simulink model "flightControlSystem"  (R2019b)
settings: Solver=ode3  StartTime=0  StopTime=TFinal  FixedStep=Ts  RelTol=1e-3  EnableMultiTasking=on
undefined symbols (not defined in the file): BINARIZER_THRESHOLD, codertarget, COG_X, COG_Y, Controller, DELAY_LANDING, DERIVATIVE_GAIN, DiscIntNeverNeededParam, Discrete, DISK_KERNEL, Estimator, FLAG_WAIT_FOR_HOVERING, FOV, FRAME_SIZE_HEIGHT, FRAME_SIZE_WIDTH, g, G_B_GAIN, GAIN_LANDING, GAIN_TRACK, gray, init, MAX_RADIUS_CROWN, MIN_RADIUS_CROWN, Sensors, SQUARE_KERNEL, strel, Time, TIME_HOLD, Ts, Vehicle, Z_HIGH, Z_LOW
libraries: simulink x37, sharedtransform x3, ctrlSharedLib x2, visionmorphops x2, sharedutil x1, parrotlib x1
(part 2 of 3)

== system flightControlSystem/Control System/Path Planning/Non linear Path Planner/Z PLANNER ==
  error_x : Inport
  flag_end_marker : Inport  Port=2
  error_y : Inport  Port=3
  flag_track : Inport  Port=4
  Chart : Stateflow chart  BlockKeywords=__PRM__SERIALIZED__DATA__:Stateflow Chart,Stateflow Diagram  TreatAsAtomicUnit=on
  Delay1 : Delay  DelayLength=DELAY_LANDING
  MATLAB Function : MATLAB Function  TreatAsAtomicUnit=on
  z_planned : Outport  VectorParamsAs1DForOutWhenUnconnected=off
  flag_end_marker_to_controller : Outport  Port=2  VectorParamsAs1DForOutWhenUnconnected=off
  wires:
  error_y/1 -> MATLAB Function/2(error_y)
  error_x/1 -> MATLAB Function/1(error_x)
  flag_end_marker/1 -> Chart/2(flag_end_marker), MATLAB Function/3(flag_end_marker)
  MATLAB Function/2(norm_error) -> Delay1/1
  Delay1/1 -> MATLAB Function/4(norm_error_prev)
  MATLAB Function/1(norm_error_tot) -> Chart/1(norm_error)
  Chart/1(z_planned) -> z_planned/1
  flag_track/1 -> Chart/3(flag_track)
  Chart/2(flag_end_marker_to_controller) -> flag_end_marker_to_controller/1

== system flightControlSystem/Control System/State Estimator/Complementary Filter/If Action Subsystem ==
  rpy : Inport
  accel : Inport  Port=2
  Action Port : ActionPort  ActionPortLabel=if(u1 > 0)
  Demux : Demux  Outputs=3
  Demux1 : Demux  Outputs=3
  Divide : Product  Inputs=*/
  Gain : Gain  Gain=1-Estimator.gyroAngleUpdateAccWeight
  Gain1 : Gain  Gain=Estimator.gyroAngleUpdateAccWeight
  Gain2 : Gain  Gain=1/g
  Gain3 : Gain  Gain=Estimator.gyroAngleUpdateAccWeight
  Gain4 : Gain  Gain=1-Estimator.gyroAngleUpdateAccWeight
  Mux : Mux  Inputs=2
  Sum : Sum  Inputs=|++
  Sum1 : Sum  Inputs=|++
  Terminator1 : Terminator
  Trigonometric Function : Trigonometry  Operator=atan
  Trigonometric Function1 : Trigonometry  Operator=asin
  pitch,roll : Outport  VectorParamsAs1DForOutWhenUnconnected=off
  wires:
  accel/1 -> Demux/1
  Demux/2 -> Divide/1
  Demux/3 -> Divide/2
  Divide/1 -> Trigonometric Function/1
  Gain/1 -> Sum/1
  Trigonometric Function/1 -> Gain1/1
  Mux/1 -> pitch,roll/1
  Gain2/1 -> Trigonometric Function1/1
  Trigonometric Function1/1 -> Gain3/1
  Gain4/1 -> Sum1/1
  Gain3/1 -> Sum1/2
  Sum1/1 -> Mux/1
  Sum/1 -> Mux/2
  rpy/1 -> Demux1/1
  Demux1/1 -> Gain/1
  Demux1/2 -> Gain4/1
  Demux/1 -> Gain2/1
  Demux1/3 -> Terminator1/1
  Gain1/1 -> Sum/2

== system flightControlSystem/Control System/State Estimator/Complementary Filter/If Action Subsystem2 ==
  prin : Inport
  Action Port : ActionPort  ActionPortLabel=else
  prout : Outport  VectorParamsAs1DForOutWhenUnconnected=off
  wires:
  prin/1 -> prout/1

== system flightControlSystem/Control System/State Estimator/Complementary Filter/Wbe ==
  rpy : Inport  OutDataTypeStr=single
  Constant : Constant  Value=single(0)
  Create 3x3 Matrix : sharedutil/Create 3x3 Matrix  aMode=aMode
  Divide : Product  Inputs=*/
  Gain : Gain  Gain=-1
  Product{1..4} (4 alike) : Product
  Selector : Selector  InputPortWidth=3  IndexOptions=Index vector (dialog)  Indices=[1]  OutputSizes=1
  Selector1 : Selector  InputPortWidth=3  IndexOptions=Index vector (dialog)  Indices=[1]  OutputSizes=1
  Selector2 : Selector  InputPortWidth=3  IndexOptions=Index vector (dialog)  Indices=[2]  OutputSizes=1
  Selector3 : Selector  InputPortWidth=3  IndexOptions=Index vector (dialog)  Indices=[2]  OutputSizes=1
  Trigonometric Function : Trigonometry  Operator=sincos
  Wbe : Outport  VectorParamsAs1DForOutWhenUnconnected=off
  wires:
  Create 3x3 Matrix/1 -> Divide/1
  Product3/1 -> Create 3x3 Matrix/8
  Trigonometric Function/2 -> Selector1/1, Selector2/1
  Selector3/1 -> Product4/2, Product3/2
  Selector1/1 -> Product4/1, Product1/1, Create 3x3 Matrix/3
  Trigonometric Function/1 -> Selector3/1, Selector/1
  Product1/1 -> Create 3x3 Matrix/5
  Product2/1 -> Create 3x3 Matrix/6
  Selector2/1 -> Divide/2, Create 3x3 Matrix/7, Product2/1, Product1/2
  Gain/1 -> Product2/2
  Product4/1 -> Create 3x3 Matrix/9
  Constant/1 -> Create 3x3 Matrix/4, Create 3x3 Matrix/1
  Divide/1 -> Wbe/1
  rpy/1 -> Trigonometric Function/1
  Selector/1 -> Product3/1, Gain/1, Create 3x3 Matrix/2

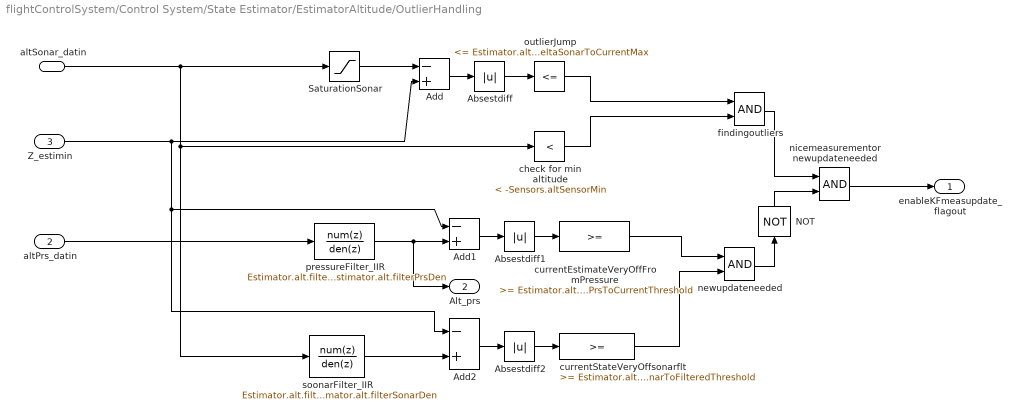
== system flightControlSystem/Control System/State Estimator/EstimatorAltitude/OutlierHandling ==
  altSonar_datin : Inport
  altPrs_datin : Inport  Port=2
  Z_estimin : Inport  Port=3
  Absestdiff : Abs
  Absestdiff1 : Abs
  Absestdiff2 : Abs
  Add : Sum  Inputs=-+
  Add1 : Sum  Inputs=-+
  Add2 : Sum  Inputs=-+
  NOT : Logic  Operator=NOT  IconShape=distinctive  AllPortsSameDT=off  OutDataTypeStr=boolean
  SaturationSonar : Saturate  UpperLimit=-Sensors.altSensorMin  LowerLimit=-inf
  check for min altitude : simulink/Logic and Bit Operations/Compare To Constant  relop=<  const=-Sensors.altSensorMin  OutDataTypeStr=boolean
  currentEstimateVeryOffFromPressure : simulink/Logic and Bit Operations/Compare To Constant  relop=>=  const=Estimator.alt.deltaPrsToCurrentThreshold  OutDataTypeStr=boolean
  currentStateVeryOffsonarflt : simulink/Logic and Bit Operations/Compare To Constant  relop=>=  const=Estimator.alt.deltaSonarToFilteredThreshold  OutDataTypeStr=boolean
  findingoutliers : Logic  AllPortsSameDT=off  OutDataTypeStr=boolean
  newupdateneeded : Logic  AllPortsSameDT=off  OutDataTypeStr=boolean
  nicemeasurementor newupdateneeded : Logic  AllPortsSameDT=off  OutDataTypeStr=boolean
  outlierJump : simulink/Logic and Bit Operations/Compare To Constant  relop=<=  const=Estimator.alt.deltaSonarToCurrentMax  OutDataTypeStr=boolean
  pressureFilter_IIR : DiscreteFilter  Numerator=Estimator.alt.filterPrsNum  Denominator=Estimator.alt.filterPrsDen
  soonarFilter_IIR : DiscreteFilter  Numerator=Estimator.alt.filterSonarNum  Denominator=Estimator.alt.filterSonarDen
  enableKFmeasupdate_flagout : Outport  VectorParamsAs1DForOutWhenUnconnected=off
  Alt_prs : Outport  Port=2  VectorParamsAs1DForOutWhenUnconnected=off
  wires:
  Add1/1 -> Absestdiff1/1
  nicemeasurementor newupdateneeded/1 -> enableKFmeasupdate_flagout/1
  findingoutliers/1 -> nicemeasurementor newupdateneeded/1
  check for min altitude/1 -> findingoutliers/2
  outlierJump/1 -> findingoutliers/1
  SaturationSonar/1 -> Add/1
  Absestdiff/1 -> outlierJump/1
  Add/1 -> Absestdiff/1
  newupdateneeded/1 -> NOT/1
  Absestdiff2/1 -> currentStateVeryOffsonarflt/1
  altSonar_datin/1 -> SaturationSonar/1, soonarFilter_IIR/1, check for min altitude/1
  currentEstimateVeryOffFromPressure/1 -> newupdateneeded/1
  Z_estimin/1 -> Add1/1, Add2/1, Add/2
  Add2/1 -> Absestdiff2/1
  currentStateVeryOffsonarflt/1 -> newupdateneeded/2
  pressureFilter_IIR/1 -> Alt_prs/1, Add1/2
  altPrs_datin/1 -> pressureFilter_IIR/1
  soonarFilter_IIR/1 -> Add2/2
  Absestdiff1/1 -> currentEstimateVeryOffFromPressure/1
  NOT/1 -> nicemeasurementor newupdateneeded/2

== system flightControlSystem/Control System/State Estimator/EstimatorXYPosition/EstimatorVelocity ==
  opticalFlow_datin : Inport
  Z_estimin : Inport  Port=2  SampleTime=Ts
  sensorIMU_datin : Inport  Port=3
  orient_estimin : Inport  Port=4
  " " : Product  Inputs=**
  AccelerationHandling : Subsystem
  Compare To Constant : simulink/Logic and Bit Operations/Compare To Constant  relop=<  const=200*4  OutDataTypeStr=boolean
  Counter Free-Running : simulink/Sources/Counter Free-Running  NumBits=32  tsamp=-1
  DataHandling : Subsystem
  Delay : Delay  DelayLength=1  InitialCondition=0
  Gain : Gain  Gain=-1
  KalmanFilter_dxdy : ctrlSharedLib/Kalman Filter  TimeDomain=Discrete-Time  UseCurrentEstimator=on  ModelSource=Individual A, B, C, D matrices  ModelSourceVariable=ss(0.95,1,1,0,1)  A=eye(2)  B=Ts*eye(2)  C=eye(2)  D=0  NumberOfStates=1  NumberOfInputs=1  NumberOfOutputs=1  InitialEstimateSource=Dialog  X0=0  P0=10  UseK=off  UseGH=on  NumberOfProcessNoiseInputs=1  G=Estimator.pos.kfVelo.G  TimeInvariantG=on  H=Estimator.pos.kfVelo.H  TimeInvariantH=on  Q=Estimator.pos.kfVelo.Q  TimeInvariantQ=on  R=Estimator.pos.kfVelo.R  TimeInvariantR=on  N=Estimator.pos.kfVelo.N  TimeInvariantN=on  AddInputPort=on  AddEnablePort=on  OutputEstimatedY=off  OutputP=off  Ts=-1
      settings: SourceProductBaseCode=CT
  Select dxy : Selector  InputPortWidth=3  IndexOptions=Index vector (dialog)  Indices=[1 2]  OutputSizes=1
  Switch : Switch  Criteria=u2 > Threshold
  Z_estimin1 : InportShadow  Port=2  SampleTime=Ts
  opticalFlowErrorCorrect : Gain  Gain=1.15
  dxy_estimout : Outport  VectorParamsAs1DForOutWhenUnconnected=off
  wires:
  Delay/1 -> DataHandling/5(dxyOF_datin)
  Z_estimin/1 -> DataHandling/1(Z_estimin), AccelerationHandling/4(Z_estimin)
  KalmanFilter_dxdy/1 -> dxy_estimout/1, Delay/1
  sensorIMU_datin/1 -> AccelerationHandling/2(sensorIMU_datin), DataHandling/3(sensorIMU_datin)
  orient_estimin/1 -> AccelerationHandling/3(orient_estimin), DataHandling/2(orient_estimin)
  Select dxy/1 -> KalmanFilter_dxdy/2, AccelerationHandling/1(dxy_estimin), DataHandling/4(dxy_estimin)
  AccelerationHandling/1(acceleration_world) -> KalmanFilter_dxdy/1
  DataHandling/1(enable_flag) -> KalmanFilter_dxdy/3
  Switch/1 -> Select dxy/1
  " "/1 -> opticalFlowErrorCorrect/1
  Gain/1 -> " "/2
  opticalFlowErrorCorrect/1 -> Switch/3
  Compare To Constant/1 -> Switch/2
  opticalFlow_datin/1 -> " "/1, Switch/1
  Z_estimin1/1 -> Gain/1
  Counter Free-Running/1 -> Compare To Constant/1

== system flightControlSystem/Control System/State Estimator/EstimatorXYPosition/EstimatorXYPosition ==
  note: Switching from orientationControl to Position
      | control reset the current world position estimate
      | (happens when using no markers)
  dxy_estimin : Inport
  orient_estimin : Inport  Port=2  SampleTime=Ts
  controlModePosVSOrient_flagin : Inport  Port=3
  dz_estimin : Inport  Port=4
  Math Function : Math  Operator=transpose  SaturateOnIntegerOverflow=on
  Mux2 : Mux  Inputs=2
  Product : Product  Multiplication=Matrix(*)
  Rotation Angles to Direction Cosine Matrix : sharedtransform/Rotation Angles to Direction Cosine Matrix  rotationOrder=ZYX  aMode=aMode
      settings: SourceProductBaseCode=AE
  SelectdXY : Selector  InputPortWidth=3  IndexOptions=Index vector (dialog)  Indices=[1 2]  OutputSizes=1
  SimplyIntegrateVelocity : DiscreteIntegrator  ExternalReset=rising  SampleTime=Ts  ICPrevOutput=DiscIntNeverNeededParam  ICPrevScaledInput=DiscIntNeverNeededParam
  XY_estimout : Outport  VectorParamsAs1DForOutWhenUnconnected=off
  wires:
  controlModePosVSOrient_flagin/1 -> SimplyIntegrateVelocity/2
  Product/1 -> SelectdXY/1
  Mux2/1 -> Product/2
  dz_estimin/1 -> Mux2/2
  SimplyIntegrateVelocity/1 -> XY_estimout/1
  dxy_estimin/1 -> Mux2/1
  orient_estimin/1 -> Rotation Angles to Direction Cosine Matrix/1
  Rotation Angles to Direction Cosine Matrix/1 -> Math Function/1
  SelectdXY/1 -> SimplyIntegrateVelocity/1
  Math Function/1 -> Product/1

== system flightControlSystem/Control System/State Estimator/SensorPreprocessing/sensordata_group ==
  HAL_acc_SI : Inport  OutDataTypeStr=Bus: HAL_acc_SI_t
  HAL_gyro_SI : Inport  Port=2  OutDataTypeStr=Bus: HAL_gyro_SI_t
  HAL_ultrasound_SI : Inport  Port=3  OutDataTypeStr=Bus: HAL_ultrasound_SI_t
  HAL_pressure_SI : Inport  Port=4  OutDataTypeStr=Bus: HAL_pressure_SI_t
  HAL_vbat_SI : Inport  Port=5  OutDataTypeStr=Bus: HAL_vbat_SI_t
  Bus Selector1 : BusSelector  OutputSignals=vbat_V,vbat_percentage
  Bus Selector3 : BusSelector  OutputSignals=x,y,z
  Bus Selector4 : BusSelector  OutputSignals=x,y,z
  Bus Selector5 : BusSelector  OutputSignals=altitude
  Bus Selector6 : BusSelector  OutputSignals=pressure
  Out Bus Element : Outport  VectorParamsAs1DForOutWhenUnconnected=off  PortName=sensordata_datin  Element=ddx
  Out Bus Element1 : Outport  VectorParamsAs1DForOutWhenUnconnected=off  PortName=sensordata_datin  Element=ddy
  Out Bus Element2 : Outport  VectorParamsAs1DForOutWhenUnconnected=off  PortName=sensordata_datin  Element=ddz
  Out Bus Element3 : Outport  VectorParamsAs1DForOutWhenUnconnected=off  PortName=sensordata_datin  Element=p
  Out Bus Element4 : Outport  VectorParamsAs1DForOutWhenUnconnected=off  PortName=sensordata_datin  Element=q
  Out Bus Element5 : Outport  VectorParamsAs1DForOutWhenUnconnected=off  PortName=sensordata_datin  Element=r
  Out Bus Element6 : Outport  VectorParamsAs1DForOutWhenUnconnected=off  PortName=sensordata_datin  Element=altitude_sonar
  Out Bus Element7 : Outport  VectorParamsAs1DForOutWhenUnconnected=off  PortName=sensordata_datin  Element=prs
  Out Bus Element8 : Outport  VectorParamsAs1DForOutWhenUnconnected=off  PortName=sensordata_datin  Element=vbat_V
  Out Bus Element9 : Outport  VectorParamsAs1DForOutWhenUnconnected=off  PortName=sensordata_datin  Element=vbat_percentage
  wires:
  HAL_gyro_SI/1 -> Bus Selector4/1
  HAL_acc_SI/1 -> Bus Selector3/1
  HAL_pressure_SI/1 -> Bus Selector6/1
  HAL_ultrasound_SI/1 -> Bus Selector5/1
  Bus Selector4/1 -> Out Bus Element3/1  "<x>"
  Bus Selector3/3 -> Out Bus Element2/1  "<z>"
  Bus Selector4/3 -> Out Bus Element5/1  "<z>"
  Bus Selector5/1 -> Out Bus Element6/1  "<altitude>"
  Bus Selector6/1 -> Out Bus Element7/1  "<pressure>"
  Bus Selector4/2 -> Out Bus Element4/1  "<y>"
  Bus Selector3/1 -> Out Bus Element/1  "<x>"
  Bus Selector3/2 -> Out Bus Element1/1  "<y>"
  Bus Selector1/1 -> Out Bus Element8/1  "<vbat_V>"
  HAL_vbat_SI/1 -> Bus Selector1/1
  Bus Selector1/2 -> Out Bus Element9/1  "<vbat_percentage>"

== system flightControlSystem/Control System/Path Planning/Non linear Path Planner/X_PLANNER/x_derivative_contribute  ==
  error_x : Inport
  Delay : Delay  DelayLength=1  InitialCondition=0
  Delay5 : Delay  DelayLength=1
  Delay6 : Delay  DelayLength=1  InitialCondition=0
  Discrete Derivative : simulink/Discrete/Discrete Derivative  gainval=Ts  ICPrevScaledInput=0.0  OutMin=[]  OutMax=[]  OutDataType=fixdt(1, 16)  OutScaling=2^-10  DoSatur=off
  MATLAB Function : MATLAB Function  TreatAsAtomicUnit=on
  derivative error : MATLAB Function  TreatAsAtomicUnit=on
  derivative_x_part : Outport  VectorParamsAs1DForOutWhenUnconnected=off
  wires:
  error_x/1 -> Discrete Derivative/1
  derivative error/3(flag_count) -> Delay5/1
  derivative error/2(count) -> Delay/1
  Delay/1 -> derivative error/4(count_prev)
  Discrete Derivative/1 -> derivative error/2(derivative_error), MATLAB Function/1(derivative_error)
  Delay5/1 -> derivative error/5(flag_count_prev)
  MATLAB Function/1(flag_change_error) -> derivative error/3(flag_change_error)
  derivative error/1(dev_contribute) -> Delay6/1, derivative_x_part/1
  Delay6/1 -> derivative error/1(dev_contribute_prev)

== system flightControlSystem/Control System/Path Planning/Non linear Path Planner/Y_PLANNER/y_derivative_contribute  ==
  error_y : Inport
  Delay : Delay  DelayLength=1  InitialCondition=0
  Delay5 : Delay  DelayLength=1
  Delay6 : Delay  DelayLength=1  InitialCondition=0
  Discrete Derivative : simulink/Discrete/Discrete Derivative  gainval=Ts  ICPrevScaledInput=0.0  OutMin=[]  OutMax=[]  OutDataType=fixdt(1, 16)  OutScaling=2^-10  DoSatur=off
  MATLAB Function : MATLAB Function  TreatAsAtomicUnit=on
  derivative error : MATLAB Function  TreatAsAtomicUnit=on
  derivative_y_part : Outport  VectorParamsAs1DForOutWhenUnconnected=off
  wires:
  error_y/1 -> Discrete Derivative/1
  derivative error/3(flag_count) -> Delay5/1
  derivative error/2(count) -> Delay/1
  Delay/1 -> derivative error/4(count_prev)
  Discrete Derivative/1 -> derivative error/2(derivative_error), MATLAB Function/1(derivative_error)
  Delay5/1 -> derivative error/5(flag_count_prev)
  MATLAB Function/1(flag_change_error) -> derivative error/3(flag_change_error)
  derivative error/1(dev_contribute) -> Delay6/1, derivative_y_part/1
  Delay6/1 -> derivative error/1(dev_contribute_prev)

== system flightControlSystem/Control System/State Estimator/EstimatorXYPosition/EstimatorVelocity/AccelerationHandling ==
  dxy_estimin : Inport
  sensorIMU_datin : Inport  Port=2
  orient_estimin : Inport  Port=3
  Z_estimin : Inport  Port=4
  Add : Sum  Inputs=-+
  Bus Selector1 : BusSelector  OutputSignals=ddx,ddy,ddz
  Deactivate Acceleration If OF is not used due to low altitude : simulink/Logic and Bit Operations/Compare To Constant  relop=<=  const=Estimator.pos.opticalFlowZMax  OutDataTypeStr=boolean
  Logical Operator : Logic  Operator=OR  AllPortsSameDT=off  OutDataTypeStr=boolean
  Mux6 : Mux  Inputs=3
  Product : Product  Inputs=3
  Product1 : Product  Multiplication=Matrix(*)
  Rotation Angles to Direction Cosine Matrix : sharedtransform/Rotation Angles to Direction Cosine Matrix  rotationOrder=ZYX  aMode=aMode
      settings: SourceProductBaseCode=AE
  SelectPlanarddxy : Selector  InputPortWidth=3  IndexOptions=Index vector (dialog)  Indices=[1 2]  OutputSizes=1
  Selector : Selector  InputPortWidth=2  IndexOptions=Index vector (dialog)  Indices=1  OutputSizes=1
  Selector1 : Selector  InputPortWidth=2  IndexOptions=Index vector (dialog)  Indices=2  OutputSizes=1
  do not use acc if optical flow never available (Note OF@60Hz but ZOH to 200!) : simulink/Logic and Bit Operations/Compare To Constant  relop=~=  const=0  OutDataTypeStr=boolean
  do not use acc if optical flow never available (Note OF@60Hz but ZOH to 200!)1 : simulink/Logic and Bit Operations/Compare To Constant  relop=~=  const=0  OutDataTypeStr=boolean
  gainaccinput : Gain  Gain=Estimator.pos.accelerationInputGain  OutDataTypeStr=single
  gravity : Constant  Value=[0 0 -g]
  acceleration_world : Outport  OutDataTypeStr=single  VectorParamsAs1DForOutWhenUnconnected=off
  wires:
  do not use acc if optical flow never available (Note OF@60Hz but ZOH to 200!)1/1 -> Logical Operator/2
  do not use acc if optical flow never available (Note OF@60Hz but ZOH to 200!)/1 -> Logical Operator/1
  Logical Operator/1 -> Product/1
  Selector1/1 -> do not use acc if optical flow never available (Note OF@60Hz but ZOH to 200!)1/1
  Selector/1 -> do not use acc if optical flow never available (Note OF@60Hz but ZOH to 200!)/1
  dxy_estimin/1 -> Selector1/1, Selector/1
  Product/1 -> acceleration_world/1
  Deactivate Acceleration If OF is not used due to low altitude/1 -> Product/3
  Z_estimin/1 -> Deactivate Acceleration If OF is not used due to low altitude/1
  Add/1 -> SelectPlanarddxy/1
  Product1/1 -> Add/1
  gravity/1 -> Product1/2
  gainaccinput/1 -> Product/2
  SelectPlanarddxy/1 -> gainaccinput/1
  Bus Selector1/3 -> Mux6/3  "<ddz>"
  Bus Selector1/1 -> Mux6/1  "<ddx>"
  sensorIMU_datin/1 -> Bus Selector1/1
  Mux6/1 -> Add/2
  Bus Selector1/2 -> Mux6/2  "<ddy>"
  orient_estimin/1 -> Rotation Angles to Direction Cosine Matrix/1
  Rotation Angles to Direction Cosine Matrix/1 -> Product1/1

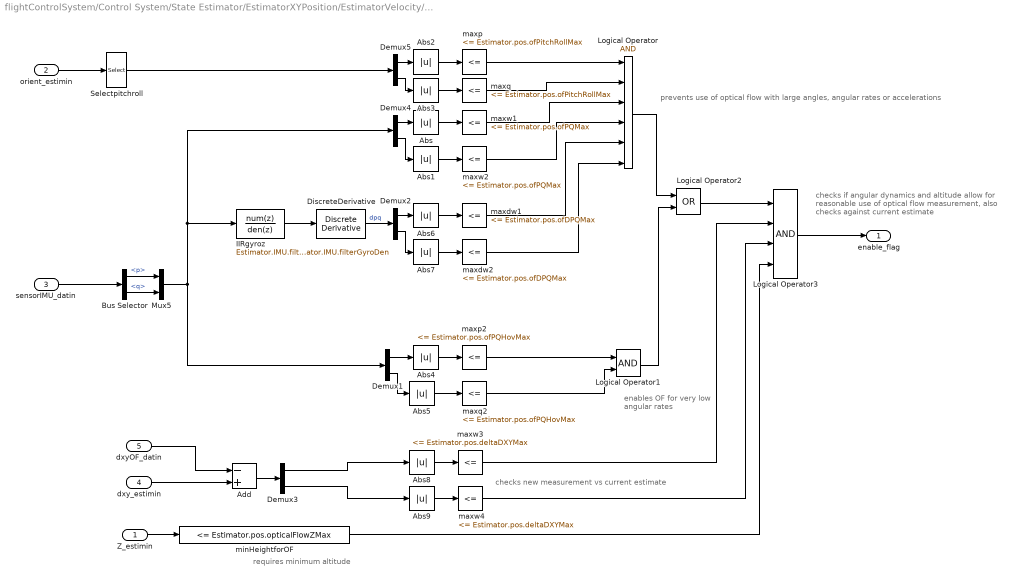
== system flightControlSystem/Control System/State Estimator/EstimatorXYPosition/EstimatorVelocity/DataHandling ==
  note: prevents use of optical flow with large angles, angular rates or accelerations
  note: enables OF for very
      | low angular rates
  note: checks if angular dynamics and altitude allow for
      | reasonable use of optical flow measurement,
      | also checks against current estimate
  note: checks new measurement vs current estimate
  note: requires minimum altitude
  Z_estimin : Inport
  orient_estimin : Inport  Port=2
  sensorIMU_datin : Inport  Port=3
  dxy_estimin : Inport  Port=4
  dxyOF_datin : Inport  Port=5
  Abs{,1..9} (10 alike) : Abs
  Add : Sum  Inputs=-+
  Bus Selector : BusSelector  OutputSignals=p,q
  Demux{1..5} (5 alike) : Demux  Outputs=2
  DiscreteDerivative : simulink/Discrete/Discrete Derivative  gainval=1.0  ICPrevScaledInput=0.0  OutMin=[]  OutMax=[]  OutDataType=fixdt(1, 16)  OutScaling=2^-10  DoSatur=off
  IIRgyroz : DiscreteFilter  Numerator=Estimator.IMU.filterGyroNum  Denominator=Estimator.IMU.filterGyroDen
  Logical Operator : Logic  Inputs=6  AllPortsSameDT=off  OutDataTypeStr=boolean
  Logical Operator1 : Logic  AllPortsSameDT=off  OutDataTypeStr=boolean
  Logical Operator2 : Logic  Operator=OR  AllPortsSameDT=off  OutDataTypeStr=boolean
  Logical Operator3 : Logic  Inputs=4  AllPortsSameDT=off  OutDataTypeStr=boolean
  Mux5 : Mux  Inputs=2
  Selectpitchroll : Selector  InputPortWidth=3  IndexOptions=Index vector (dialog)  Indices=[2 3]  OutputSizes=1
  maxdw1 : simulink/Logic and Bit Operations/Compare To Constant  relop=<=  const=Estimator.pos.ofDPQMax  OutDataTypeStr=boolean
  maxdw2 : simulink/Logic and Bit Operations/Compare To Constant  relop=<=  const=Estimator.pos.ofDPQMax  OutDataTypeStr=boolean
  maxp : simulink/Logic and Bit Operations/Compare To Constant  relop=<=  const=Estimator.pos.ofPitchRollMax  OutDataTypeStr=boolean
  maxp2 : simulink/Logic and Bit Operations/Compare To Constant  relop=<=  const=Estimator.pos.ofPQHovMax  OutDataTypeStr=boolean
  maxq : simulink/Logic and Bit Operations/Compare To Constant  relop=<=  const=Estimator.pos.ofPitchRollMax  OutDataTypeStr=boolean
  maxq2 : simulink/Logic and Bit Operations/Compare To Constant  relop=<=  const=Estimator.pos.ofPQHovMax  OutDataTypeStr=boolean
  maxw1 : simulink/Logic and Bit Operations/Compare To Constant  relop=<=  const=Estimator.pos.ofPQMax  OutDataTypeStr=boolean
  maxw2 : simulink/Logic and Bit Operations/Compare To Constant  relop=<=  const=Estimator.pos.ofPQMax  OutDataTypeStr=boolean
  maxw3 : simulink/Logic and Bit Operations/Compare To Constant  relop=<=  const=Estimator.pos.deltaDXYMax  OutDataTypeStr=boolean
  maxw4 : simulink/Logic and Bit Operations/Compare To Constant  relop=<=  const=Estimator.pos.deltaDXYMax  OutDataTypeStr=boolean
  minHeightforOF : simulink/Logic and Bit Operations/Compare To Constant  relop=<=  const=Estimator.pos.opticalFlowZMax  OutDataTypeStr=boolean
  enable_flag : Outport  VectorParamsAs1DForOutWhenUnconnected=off
  wires:
  minHeightforOF/1 -> Logical Operator3/4
  IIRgyroz/1 -> DiscreteDerivative/1
  Mux5/1 -> Demux1/1, IIRgyroz/1, Demux4/1
  maxw4/1 -> Logical Operator3/3
  maxw3/1 -> Logical Operator3/2
  dxyOF_datin/1 -> Add/1
  Demux3/2 -> Abs9/1
  Demux3/1 -> Abs8/1
  dxy_estimin/1 -> Add/2
  Add/1 -> Demux3/1
  Abs9/1 -> maxw4/1
  Abs8/1 -> maxw3/1
  Logical Operator2/1 -> Logical Operator3/1
  Logical Operator3/1 -> enable_flag/1
  DiscreteDerivative/1 -> Demux2/1  "dpq"
  Demux2/2 -> Abs7/1
  Demux2/1 -> Abs6/1
  Abs7/1 -> maxdw2/1
  Abs6/1 -> maxdw1/1
  Logical Operator1/1 -> Logical Operator2/2
  Demux1/2 -> Abs5/1
  Demux1/1 -> Abs4/1
  Abs5/1 -> maxq2/1
  Abs4/1 -> maxp2/1
  Abs3/1 -> maxq/1
  Abs2/1 -> maxp/1
  Demux4/2 -> Abs1/1
  Demux4/1 -> Abs/1
  Abs1/1 -> maxw2/1
  Abs/1 -> maxw1/1
  Z_estimin/1 -> minHeightforOF/1
  Logical Operator/1 -> Logical Operator2/1
  maxw1/1 -> Logical Operator/3
  Bus Selector/1 -> Mux5/1  "<p>"
  Selectpitchroll/1 -> Demux5/1
  sensorIMU_datin/1 -> Bus Selector/1
  maxq2/1 -> Logical Operator1/2
  Bus Selector/2 -> Mux5/2  "<q>"
  maxp/1 -> Logical Operator/1
  maxw2/1 -> Logical Operator/4
  orient_estimin/1 -> Selectpitchroll/1
  maxdw1/1 -> Logical Operator/5
  maxdw2/1 -> Logical Operator/6
  maxq/1 -> Logical Operator/2
  Demux5/1 -> Abs2/1
  Demux5/2 -> Abs3/1
  maxp2/1 -> Logical Operator1/1

== matlab function flightControlSystem/Control System/Path Planning/Non linear Path Planner/X_PLANNER/x_derivative_contribute /derivative error ==
  data: dev_contribute_prev input; derivative_error input; flag_change_error input; dev_contribute output; count_prev input; count output; flag_count_prev input; flag_count output; Ts parameter; TIME_HOLD parameter; DERIVATIVE_GAIN parameter
function [dev_contribute, count, flag_count] = derivative_error(dev_contribute_prev, ...
    derivative_error, flag_change_error,count_prev,flag_count_prev, Ts, ...
    TIME_HOLD, DERIVATIVE_GAIN)
% This MATLAB function computes the derivative contribution of the path planner
% for the x coordinate.
%
% Inputs:
% - dev_contribute_prev: previous value derative part of the planner
% - derivative_error: derivative error value.
% - flag_change_error: it is raised when the sign of the error changes
% - count_prev: previous value of the counter. 
%
% Parameters:
% - Ts: sampling Time.
% - TIME_HOLD: time to which the previous value assumed by the derivative
% contribute has to be hold.
% - DERIVATIVE_GAIN: gain used for the derivative contribution.
%
% Output:
% - dev_contribute: derivative contribution of the path planner.
% - count: counter value
% - flag_count: flag raises when the derivate contribute does not more take
% part to the pat planner.

persistent count_to_be_hold

if isempty(count_to_be_hold)
    count_to_be_hold = round(TIME_HOLD/Ts);
end

flag_count = 0;

if flag_change_error && count_prev == 0    
    flag_count=1;   
end
   
if flag_count_prev || flag_count
    
    if count_prev == count_to_be_hold

        count=0;
        flag_count=0;

    else

        count=count_prev+1;
        flag_count=1;
        
    end
    
    dev_contribute=derivative_error*DERIVATIVE_GAIN;
    
    if dev_contribute ==0 && dev_contribute_prev ~=0 
        
        dev_contribute=dev_contribute_prev;
        
    end

else
    
    flag_count = 0;
    count = 0;
    dev_contribute = 0;
    
end

== matlab function flightControlSystem/Control System/Path Planning/Take off Checker ==
  data: flag_activate_PP output; z_est input; Z_LOW parameter; Z_HIGH parameter; FLAG_WAIT_FOR_HOVERING parameter
function flag_activate_PP = height_checker(z_est, Z_LOW, Z_HIGH, FLAG_WAIT_FOR_HOVERING)
% This MATLAB function raise a flag when the drone is hovering by using the
% z_low and z_high variable which are threshold level expressed in meters. The output is a
% flag that permits the path planner to be activated and perform the
% trajectory tracking.
%
% Inputs:
% - z_low: low threshold height, in meters
% - z_high: high threshold height, in meters
% - z_est: estimation of drone's height 
% - FLAG_WAIT_FOR_HOVERING: the flag is used to decide if path planner is
% activie before or after drone takes off (TRUE/FALSE)
%
% Output:
% - flag_activate_PP: the flag is used to activate the Path Planner.

if FLAG_WAIT_FOR_HOVERING == 0
    
    if z_est < Z_LOW && z_est > Z_HIGH
        
        flag_activate_PP = 1 ;
    else
        
        flag_activate_PP = 0 ;
        
    end
    
else
    
    flag_activate_PP = 1 ;
    
end

end

== matlab function flightControlSystem/Control System/Path Planning/MATLAB Function ==
  data: x_err_tr input; x_error output; y_err_tr input; x_err_ea input; y_err_ea input; flag_ea input; flag_ho input; y_error output
function [x_error, y_error] = decision_making(x_err_tr, y_err_tr, x_err_ea, ...
    y_err_ea, flag_ea, flag_ho)
% The MALTAB function sends the error along x- and y-axis to the drone 
% trajectory controller. When the "flag_ea" is low, the position errors
% are computed as the difference between the end-marker and the drone
% CoG. Instead, when the flag is high, the errors are computed by the
% Image Processing System.
%
% Inputs:
% - x_err_tr: tracking error along the x-axis. The error is expressed in 
% pixels.
% - y_err_tr: tracking error along the y-axis. The error is expressed in 
% pixels.
% - x_err_ea: position error along the x-axis when the end-marker is 
% detected. The error is expressed in pixels.
% - y_err_ea: position error along the y-axis when the end-marker is
% detected. The error is expressed in pixels.
% - flag_ea: the flag allows to check if the end-maker is recognized.
% - flag_ho: the flag allows to check if the drone is able to fly.
%   
% Outputs
% - x_error: error between the drone CoG and the track/end-marker along the 
% x-axis. The error is expressed in pixels.
% - y_error: error between the drone CoG and the track/end-marker along the
% y-axis. The error is expressed in pixels

if flag_ho == 1
    
    if flag_ea == 0
        
        x_error=x_err_tr;
        y_error=y_err_tr;
              
    else
        
        x_error=x_err_ea;
        y_error=y_err_ea;
        
    end
    
else
    
    x_error=0;
    y_error=0;
    
end
    
end

== matlab function flightControlSystem/Image Processing System/Waypoints Follower/waypoints 1 ==
  data: frame input; error_y_track output; error_x_track output; x_ref_prev input; y_ref_prev input; orientation_track output; flag_track output; flag_track_prev input; MIN_RADIUS_CROWN parameter; MAX_RADIUS_CROWN parameter; FOV parameter; COG_X parameter; COG_Y parameter
function [error_y_track, error_x_track, orientation_track, flag_track] = ...
error_pixel_generator(frame, x_ref_prev, y_ref_prev, flag_track_prev, ...
MIN_RADIUS_CROWN, MAX_RADIUS_CROWN, FOV, COG_X, COG_Y)
% The MATLAB function computes the error along x and y-axis between
% the drone COG (Center of Gravity) and the point of the track extract 
% by using of a crown circular mask. This errors is later used by the Path 
% Planner for the lane tracking  
%
%
% Inputs:
% - frame: binarized frame
% - x_ref_prev: previous value of the tracking point along the x-axis of 
% the track line. It is used as a reference for tracking the path.
% - y_ref_prev: previous value of the tracking point along the y-axis of 
% the track line. It is used as a reference for tracking the path.                                                                                                                                              
% - flag_track_prev: previous value assumed by the flag variablle, i.e., 
% the previous state of the drone (over the track / not over the track).
%
%
% Outputs:
% - error_y_track: error between the CoG of the drone and a point of the 
% lane in the forward direction along the y-axis. It is expressed in
% pixels.
% - error_x_track: error between the CoG of the drone and a point of the 
% lane in the forward direction along the x-axis. It is expressed in pixels. 
% - flag_track: it indicates if the drone is currently over the track (TRUE).
% - yaw: the heading angle of the track in the image plane.
%
%
% Parameters:
% - MIN_RADIUS_CROWN: minimum value of the radius of the crown mask. It is
% expressed in pixels.
% - MAX_RADIUS_CROWN: maximum value of the radius of the crown mask. It is
% expressed in pixels.
% - FOV: a portion of the crown used to detect the lane. It is expressed in
% radians.
% - COG_X: position of the drone CoG along x-axis of the reference frame.
% - COG_Y: position of the drone CoG along y-axis of the reference frame.

persistent x_accumulator
persistent y_accumulator
persistent pixel_count

if isempty(x_accumulator)
    x_accumulator = 0;
end

if isempty(y_accumulator)
    y_accumulator = 0;
end

if isempty(pixel_count)
    pixel_count = 0;
end

% the previous value of the heading angle of the lane 
orientation_track = atan2(-x_ref_prev,y_ref_prev); 
orientation_track = mod(orientation_track,2*pi);

% checking if the drone is over the lane
if flag_track_prev     

    % the set of pixels inside the crown mask
    for i = (COG_X-MAX_RADIUS_CROWN):(COG_X+MAX_RADIUS_CROWN) 

        for j = (COG_Y-MAX_RADIUS_CROWN):(COG_Y+MAX_RADIUS_CROWN)

            norm = sqrt(((i-(COG_X-0.5))^2)+((j-(COG_Y-0.5))^2));

            if norm >= MIN_RADIUS_CROWN && norm <= MAX_RADIUS_CROWN 

                axis_x = (i-(COG_X-0.5));
                axis_y = (j-(COG_Y-0.5));
                yaw_point_temp = atan2(axis_x,axis_y);


                yaw_point_temp_2 = mod(yaw_point_temp,2*pi);

                % a portion of the crown mask depending on the FOV
                threshold_1 = mod((orientation_track+(pi/FOV)),2*pi);

                threshold_2 = mod((orientation_track-(pi/FOV)),2*pi);

                if threshold_1 < threshold_2

                    flag_threshold = ...
                        (yaw_point_temp_2 <= 2*pi  && yaw_point_temp_2 >= threshold_2) ...
                        || (yaw_point_temp_2 <= threshold_1  && yaw_point_temp_2 >= 0);

                else

                    flag_threshold = ...
                        yaw_point_temp_2 <= threshold_1  && yaw_point_temp_2 >= threshold_2;

                end

                if flag_threshold
 
                    if frame(i,j)==1 
                        
                        pixel_count = pixel_count + 1;
                        x_accumulator = x_accumulator + i;
                        y_accumulator = y_accumulator + j;

                    end

                end

            end

        end
    end
    
else
    % checking for the initial heading angle of the lane. It can be 
    % different from the heading angle of the drone
    for i = (COG_X-MAX_RADIUS_CROWN):(COG_X+MAX_RADIUS_CROWN)

        for j = (COG_Y-MAX_RADIUS_CROWN):(COG_Y+MAX_RADIUS_CROWN)
            
            norm=sqrt(((i-(COG_X-0.5))^2)+((j-(COG_Y-0.5))^2));

            if norm>=MIN_RADIUS_CROWN && norm <= MAX_RADIUS_CROWN 

                axis_x = (i-(COG_X-0.5));
                axis_y = (j-(COG_Y-0.5));

                if frame(i,j)==1 
                    pixel_count=pixel_count +1;
                    x_accumulator=x_accumulator+i;
                    y_accumulator=y_accumulator+j;
                end
            end
        end
    end
end

% calculating the medium point of the lane as output of the mask
x_ref_temp = -(round(x_accumulator/pixel_count)-COG_X);
y_ref_temp = (round(y_accumulator/pixel_count)-COG_Y);

% when there is no track, the x_ref_temp and y_ref_temp variables are NaN.
% Below is the code for fix the issue.

if isnan(x_ref_temp)
    
    % if the computer vision algorithm does not detect the track, the 
    % drone position does not change
    error_x_track = 0 ;
    flag_error_x = false;
    
else
    
    % if the computer vision algorithm detects the track, a new position 
    % is computed for the tracking problem
    flag_error_x = true;
    error_x_track = x_ref_temp;
    
end

% As for the x coordinate
if isnan(y_ref_temp)
    
    error_y_track = 0 ;
    flag_error_y = false;
    
else
    
    error_y_track = y_ref_temp;
    flag_error_y=true ;
    
end

% checking if the drone is over the lane
flag_track = flag_error_x || flag_error_y;

% reset of the persistent variables
pixel_count = 0;
x_accumulator = 0;
y_accumulator = 0;

end

== matlab function flightControlSystem/Control System/Path Planning/Non linear Path Planner/Y_PLANNER/y_derivative_contribute /MATLAB Function ==
  data: derivative_error input; flag_change_error output; CHANGE_DERIVATIVE_ERROR_THRESHOLD parameter
function flag_change_error = change_error_checker(derivative_error, ...
    CHANGE_DERIVATIVE_ERROR_THRESHOLD)
% This MATLAB function recognizes if the derivative of the error is greater
% than a threshold value, i.e., the  CHANGE_DERIVATIVE_ERROR_THRESHOLD. 
% 
% Input:
% - derivative_error: derivative of the error. The error is expressed in 
% pixels
%
% Parameter:
% - CHANGE_DERIVATIVE_ERROR_THRESHOLD: threshold value.
%
% Output:
% - flag_change_error: flag raised when the derivative of the error
% changes.

if abs(derivative_error) >= CHANGE_DERIVATIVE_ERROR_THRESHOLD

    flag_change_error = 1;

else

    flag_change_error = 0;

end

== stateflow chart flightControlSystem/Control System/Path Planning/Non linear Path Planner/Z PLANNER/Chart ==
  state STATE [group]
    - TRACKING: The drone is tracking the lane or the end-marker when they are detected.
    - LANDING: The drone is landing when the land-marker is detected and the error between the drone CoG and
    the central point of the end-marker is less than MAX_ERROR_LANDING.
  state INPUT [group]
    - flag_track: flag raised when the lane is detected by the Image Processing System.
    - flag_end_marker: flag raised when the end-marker is detected by the Image Processing System.
    - norm error: error between the drone CoG and the central point of the end-marker.
  state OUTPUT [group]
    - z_planned: drone altitude sent to the drone controller.
    - flag_end_marker_to_controller: flag raise when the drone has to land.
  state TRACKING
    entry:
    z_planned =  -1.1 ;
    flag_end_marker_to_controller=0;
  state LANDING
    entry:
    z_planned =  0 ;
    flag_end_marker_to_controller=1;
  state IDLE
    entry:
    z_planned =  -1.1 ;
    flag_end_marker_to_controller=0;
  (default) -> IDLE
  IDLE -> TRACKING : [flag_track==1]
  TRACKING -> LANDING : [flag_end_marker==1 && norm_error <= MAX_ERROR_LANDING]
  data: norm_error input double; z_planned output double; MAX_ERROR_LANDING parameter double; flag_end_marker input; flag_track input; flag_end_marker_to_controller output double

== matlab function flightControlSystem/Image Processing System/Land Mark Detector ==
  data: output output; binary input; waypoint_follower_variable input; FRAME_SIZE_WIDTH parameter; FRAME_SIZE_HEIGHT parameter; COG_Y parameter; COG_X parameter
function output = end_marker_detector(binary, waypoint_follower_variable, ...
    FRAME_SIZE_WIDTH, FRAME_SIZE_HEIGHT, COG_Y, COG_X)
% The MATLAB function computes the errors along the x- and y-axis between
% the drone COG and the middle of the lane. The end marker is detected by 
% using a disk kernel. This function is active only when the drone has 
% arrived at the end of the path.
%
%
% Inputs:
% - binary: binarized frame obtained as the convolution with a disk kernel
% - x_ref_prev: previous value of the tracking point along the x-axis of 
% the track line. It is used as a reference for tracking the path.
% - y_ref_prev: previous value of the tracking point along the y-axis of 
% the track line. It is used as a reference for tracking the path. 
% - flag_track_prev: previous value assumed by the flag variablle, i.e., 
% the previous state of the drone (over the track / not over the track).
%
%
% Outputs:
% - error_y_end_marker: error between the CoG of the drone and a point of the 
% lane in the forward direction along the y-axis. It is expressed in
% pixels.
% - error_x_end_maker: error between the CoG of the drone and a point of the 
% lane in the forward direction along the x-axis. It is expressed in pixels. 
% - flag_end_marker: it is TURE if the Image Processing System detects 
% the end marker.
% - yaw: heading angle of the lane in the image plane.
%
%
%Parameters:
% - COG_X: position of the drone CoG along x-axis of the reference frame.
% - COG_Y: position of the drone CoG along y-axis of the reference frame.
% - FRAME_SIZE_WIDTH: width of the frame.
% - FRAME_SIZE_HEIGHT: height of the frame.

persistent column_accumulator
persistent count_pixel
persistent row_accumulator

if isempty(column_accumulator)
    column_accumulator = 0;
end

if isempty(count_pixel)
    count_pixel = 0;
end

if isempty(row_accumulator)
    row_accumulator = 0;
end

flag_track = waypoint_follower_variable(3);


% check if the track is ended
if ~flag_track

    for i=1:FRAME_SIZE_HEIGHT

        for j=1:FRAME_SIZE_WIDTH

            %check all the pixel belonging to the end marker
            if binary(i,j)==1
                count_pixel = count_pixel +1;
                column_accumulator = column_accumulator + j;
                row_accumulator = row_accumulator + i;

            end

        end
    end
    
    if count_pixel ~= 0
        flag_end_marker=1;
        center_x = round(row_accumulator/count_pixel);
        center_y = round(column_accumulator/count_pixel);
    else
        flag_end_marker=0;
        center_x=1;
        center_y=1;
    end

else
    
    center_x = 0;
    center_y = 0;
    flag_end_marker = 0;

end

% Calculate the medium point of the end marker
error_x_end_marker = -(center_x - COG_X);
error_y_end_marker = (center_y - COG_Y);

% reset of the persistent variables
count_pixel = 0;
column_accumulator = 0;
row_accumulator = 0;

output = [error_x_end_marker, error_y_end_marker, flag_end_marker];

end

== stateflow chart flightControlSystem/Control System/Path Planning/Non linear Path Planner/X_PLANNER/x_linear_contribute ==
  state STATE [group]
    - TRACK_DETECTED: The Image Processing System detected the lane.
    - END_MARKER_DETECTED: The Image Processing System detected the end-marker.
  state INPUT [group]
    - Flag_track: flag raised when the lane is detected by the Image Processing System.
    - Flag_end_marker : flag raised when the end-marker is detected by the Image Processing System.
  state PARAMETERS [group]
    - GAIN_TRACK: gain used from the drone reference generator when it follows the lane.
    - GAIN_LANDING: gain used from the drone reference generator for landing on the end-marker.
  state OUTPUT [group]
    - linear_part : linear contribute.
  state END_MARKER_DETECTED
    during:
    linear_part = error * GAIN_LANDING;
  state IDLE
  state TRACK_DETECTED
    during:
    linear_part = error * GAIN_TRACK;
  TRACK_DETECTED -> END_MARKER_DETECTED : [flag_end_marker==1 && flag_track==0]
  IDLE -> TRACK_DETECTED : [flag_end_marker==0 && flag_track==1]
  (default) -> IDLE
  data: error input double; GAIN_TRACK parameter double; GAIN_LANDING parameter double; flag_end_marker input double; flag_track input double; linear_part output double

== matlab function flightControlSystem/Control System/Path Planning/Non linear Path Planner/Z PLANNER/MATLAB Function ==
  data: norm_error_tot output; error_x input; norm_error output; error_y input; flag_end_marker input; norm_error_prev input
function [norm_error_tot, norm_error] = error_function(error_x, error_y, ...
flag_end_marker, norm_error_prev)
% This MATLAB function computes the norm of the error between the drone CoG
% drone and the middle of point of the end-marker. The norm error is
% computed only if the end-marker is detected.
%
%
%Inputs:
% - error_x: error along the x-axis between the drone CoG and the central 
% point of the end-marker.
% - error_y: error along the y-axis between the drone CoG and the central 
% point of the end-marker.
% - flag_end_marker: the flag indicates when the end-marker is detected.
% - norm_error_prev: previous value of the norm of the error.                                                                                                                                              
%  
%
%Outputs:
% - norm_error_tot: norm of the error between the drone CoG and the central 
% point of the end-marker. It consideres the previous value assumed by the
% norm of the error. The values is condisder at the time k = time_step +
% DELAY_LANDING \cdot sampling time. 
% - norm_error: actual value assumed by the norm of error. The error is 
% computed by the drone CoG and the middle point of the end-marker.

if flag_end_marker
    
    norm_error = sqrt((error_x)^2 + (error_y)^2);
    norm_error_tot = norm_error + norm_error_prev  ;
    
else 
    %100 is a constant value greater than MAX_ERROR_LANDING
    norm_error_tot = 100;
    norm_error = 100;
end

== matlab function flightControlSystem/Control System/Path Planning/Non linear Path Planner/Y_PLANNER/y_derivative_contribute /derivative error ==
  data: dev_contribute_prev input; derivative_error input; flag_change_error input; dev_contribute output; count_prev input; count output; flag_count_prev input; flag_count output; Ts parameter; TIME_HOLD parameter; DERIVATIVE_GAIN parameter
function [dev_contribute, count, flag_count] = derivative_error(dev_contribute_prev, ...
    derivative_error, flag_change_error,count_prev,flag_count_prev, Ts, ...
    TIME_HOLD, DERIVATIVE_GAIN)
% This MATLAB function computes the derivative contribution of the path planner
% for the x coordinate.
%
% Inputs:
% - dev_contribute_prev: previous value derative part of the planner
% - derivative_error: derivative error value.
% - flag_change_error: it is raised when the sign of the error changes
% - count_prev: previous value of the counter. 
%
% Parameters:
% - Ts: sampling Time.
% - TIME_HOLD: time to which the previous value assumed by the derivative
% contribute has to be hold.
% - DERIVATIVE_GAIN: gain used for the derivative contribution.
%
% Output:
% - dev_contribute: derivative contribution of the path planner.
% - count: counter value
% - flag_count: flag raises when the derivate contribute does not more take
% part to the pat planner.

persistent count_to_be_hold

if isempty(count_to_be_hold)
    count_to_be_hold = round(TIME_HOLD/Ts);
end

flag_count = 0;

if flag_change_error && count_prev == 0    
    flag_count=1;   
end
   
if flag_count_prev || flag_count
    
    if count_prev == count_to_be_hold

        count=0;
        flag_count=0;

    else

        count=count_prev+1;
        flag_count=1;
        
    end
    
    dev_contribute=derivative_error*DERIVATIVE_GAIN;
    
    if dev_contribute ==0 && dev_contribute_prev ~=0 
        
        dev_contribute=dev_contribute_prev;
        
    end

else
    
    flag_count = 0;
    count = 0;
    dev_contribute = 0;
    
end

== matlab function flightControlSystem/Control System/Path Planning/Non linear Path Planner/X_PLANNER/x_derivative_contribute /MATLAB Function ==
  data: derivative_error input; flag_change_error output; CHANGE_DERIVATIVE_ERROR_THRESHOLD parameter
function flag_change_error = change_error_checker(derivative_error, ...
    CHANGE_DERIVATIVE_ERROR_THRESHOLD)
% This MATLAB function recognizes if the derivative of the error is greater
% than a threshold value, i.e., the  CHANGE_DERIVATIVE_ERROR_THRESHOLD. 
% 
% Input:
% - derivative_error: derivative of the error. The error is expressed in 
% pixels
%
% Parameter:
% - CHANGE_DERIVATIVE_ERROR_THRESHOLD: threshold value.
%
% Output:
% - flag_change_error: flag raised when the derivative of the error
% changes.

if abs(derivative_error) >= CHANGE_DERIVATIVE_ERROR_THRESHOLD

    flag_change_error = 1;

else

    flag_change_error = 0;

end

== stateflow chart flightControlSystem/Control System/Path Planning/Non linear Path Planner/Y_PLANNER/Chart1 ==
  state STATE [group]
    - TRACKING: the drone is tracking the lane of the end-marker.
    - LANDING: the drone is landing when the end-marker is dected and the error between the drone CoG and the
    middle point of the end-marker is less than MAX_ERROR_LANDING.
    - TRACK_DETECTED: the Image Processing System detected the lane.
    - END_MARKER_DETECTED: the Image Processing System detected the end-marker.
  state INPUT [group]
    - flag_track: flag raised when the track is detected by Image Processing System.
    - flag_end_marker_to_Controller: flag raised when the drone has to land.
    - lin_part: linear part of the path planner.
    - dev_part: derivative part of the path planner.
    - y_estimated: estimated drone position along the y-axis.
    - flag_end_marker : flag raised when the end-marker is detected by the Image Processing System.
  state OUTPUT [group]
    - y_planned: y coordinate of the goal position.
  state TRACKING
    state TRACK_DETECTED
      during:
      y_planned= y_estimated + lin_part + dev_part;
      y_planned_stored=y_planned;
    state END_MARKER_DETECTED
      during:
      y_planned= y_estimated + lin_part ;
      y_planned_stored=y_planned;
    (default) -> TRACK_DETECTED
    TRACK_DETECTED -> END_MARKER_DETECTED : [flag_end_marker==1 && flag_track==0]
    END_MARKER_DETECTED -> TRACK_DETECTED : [flag_end_marker==0 && flag_track==1]
  state LANDING
    during:
    y_planned=y_planned_stored;
  state IDLE
  (default) -> IDLE
  IDLE -> TRACKING : [flag_track==1 && flag_end_marker==0]
  TRACKING -> LANDING : [flag_end_marker_to_controller==1]
  data: dev_part input double; lin_part input double; flag_end_marker_to_controller input double; flag_track input double; flag_end_marker input double; y_estimated input; y_planned_stored local double; y_planned output double

== stateflow chart flightControlSystem/Image Processing System/Waypoints Follower/state machine ==
  state STATE [group]
    - ON_TRACK: the Image Processing System detects the lane. The drone is on the lane.
    - END_TRACK: it indicates the end of the lane.
  state OUTPUT [group]
    - FLAG: it indicates the presence or not of the track path
  state INPUT [group]
    - FLAG_TRACK: flag raises when the track is detected from Image Processing System.
  state END_TRACK
    entry: flag=0;
  state ON_TRACK
    entry: flag=1;
  state TAKE_OFF
    entry: flag=1;
  ON_TRACK -> END_TRACK : [flag_track==0]
  TAKE_OFF -> ON_TRACK : [flag_track==1]
  (default) -> TAKE_OFF
  data: flag_track input; flag output
